simulink model "motor_sim"  (R2024a)
settings: Solver=FixedStepAuto  StartTime=0.0  StopTime=inf  FixedStep=0.0005  RelTol=1e-3
undefined symbols (not defined in the file or in its folder): B, circumference_tyre, J, K_b, K_t, L, PI, R, ratio_reduction, tau_L
libraries: canoelib x4
settings Model: Creator=user  LastModifiedBy=user

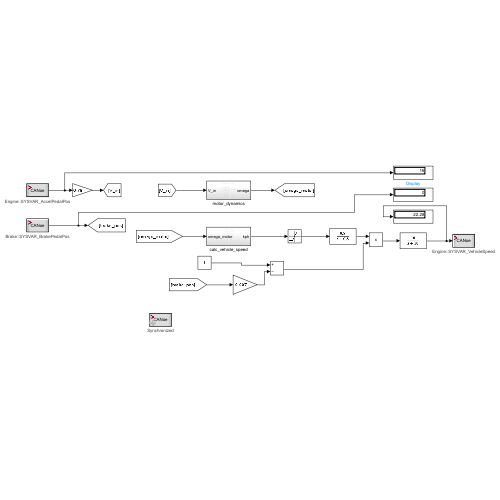
[thumbnail: Simulink's stored preview of the top-level diagram]
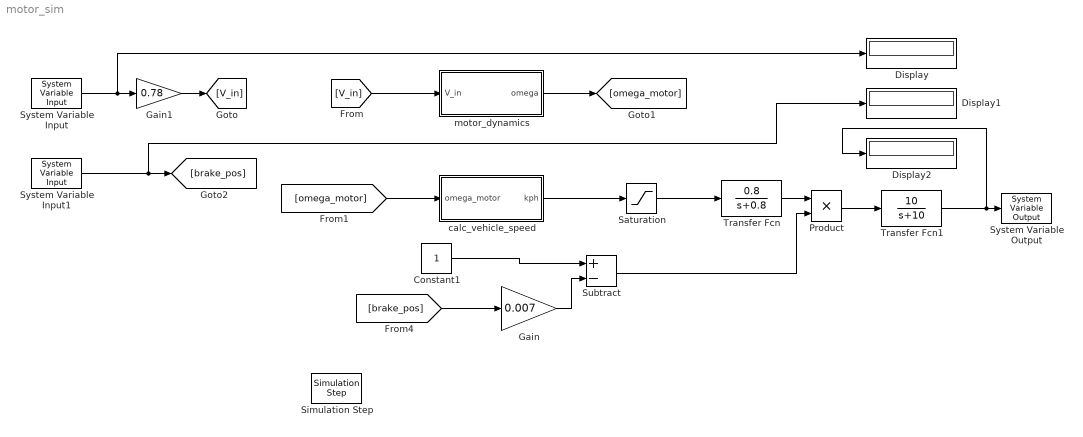
== system motor_sim ==
  Constant1 : Constant
  Display : Display
  Display1 : Display
  Display2 : Display
  Gain : Gain  Gain=0.007
  Gain1 : Gain  Gain=0.78
  Product : Product
  Saturation : Saturate  UpperLimit=250  LowerLimit=0
  Simulation Step : canoelib/CANoe I//O/Simulation Step  mode=Synchronized
      settings: AttributesFormatString=%<mode>  SourceProductName=Vector CANoe
  Subtract : Sum  Inputs=+-
  System Variable Input : canoelib/CANoe I//O/System Variable Input  nsName=Engine  sysVarName=SYSVAR_AccelPedalPos  arrayIndex=-1  editSampleTime=0  rawValue=Default  dataType=Default  dataTypeDB=uint32  hasEncoding=off  dataTypeCANoe=Get from CANoe
      settings: AttributesFormatString=%<nsName>::%<sysVarName>  SourceProductName=Vector CANoe
  System Variable Input1 : canoelib/CANoe I//O/System Variable Input  nsName=Brake  sysVarName=SYSVAR_BrakePedalPos  arrayIndex=-1  editSampleTime=0  rawValue=Default  dataType=Default  dataTypeDB=uint32  hasEncoding=off  dataTypeCANoe=Get from CANoe
      settings: AttributesFormatString=%<nsName>::%<sysVarName>  SourceProductName=Vector CANoe
  System Variable Output : canoelib/CANoe I//O/System Variable Output  nsName=Engine  sysVarName=SYSVAR_VehicleSpeed  arrayIndex=-1  rawValue=Default  dataType=Default  dataTypeDB=uint32  hasEncoding=off  dataTypeCANoe=Get from CANoe
      settings: AttributesFormatString=%<nsName>::%<sysVarName>  SourceProductName=Vector CANoe
  Transfer Fcn : TransferFcn  Numerator=[0.8]  Denominator=[1 0.8]
  Transfer Fcn1 : TransferFcn  Numerator=[10]  Denominator=[1 10]
  calc_vehicle_speed : Subsystem
  motor_dynamics : Subsystem
  wires:
  [V_in] -> motor_dynamics/1(V_in)
  motor_dynamics/1(omega) -> [omega_motor]
  calc_vehicle_speed/1(kph) -> Saturation/1
  [omega_motor] -> calc_vehicle_speed/1(omega_motor)
  [brake_pos] -> Gain/1
  Constant1/1 -> Subtract/1
  Gain/1 -> Subtract/2
  Subtract/1 -> Product/2
  Saturation/1 -> Transfer Fcn/1
  Transfer Fcn/1 -> Product/1
  Product/1 -> Transfer Fcn1/1
  System Variable Input/1 -> Display/1, Gain1/1
  Gain1/1 -> [V_in]
  System Variable Input1/1 -> Display1/1, [brake_pos]
  Transfer Fcn1/1 -> Display2/1, System Variable Output/1

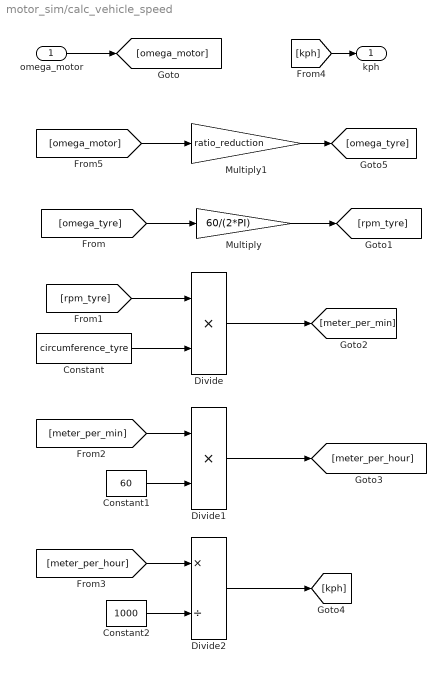
== system motor_sim/calc_vehicle_speed ==
  omega_motor : Inport
  Constant : Constant  Value=circumference_tyre
  Constant1 : Constant  Value=60
  Constant2 : Constant  Value=1000
  Divide : Product  Inputs=**
  Divide1 : Product  Inputs=**
  Divide2 : Product  Inputs=*/
  Multiply : Gain  Gain=60/(2*PI)
  Multiply1 : Gain  Gain=ratio_reduction
  kph : Outport
  wires:
  omega_motor/1 -> [omega_motor]
  [omega_tyre] -> Multiply/1
  Multiply/1 -> [rpm_tyre]
  [rpm_tyre] -> Divide/1
  Constant/1 -> Divide/2
  Divide/1 -> [meter_per_min]
  [meter_per_min] -> Divide1/1
  Constant1/1 -> Divide1/2
  Divide1/1 -> [meter_per_hour]
  [meter_per_hour] -> Divide2/1
  Constant2/1 -> Divide2/2
  Divide2/1 -> [kph]
  [kph] -> kph/1
  [omega_motor] -> Multiply1/1
  Multiply1/1 -> [omega_tyre]

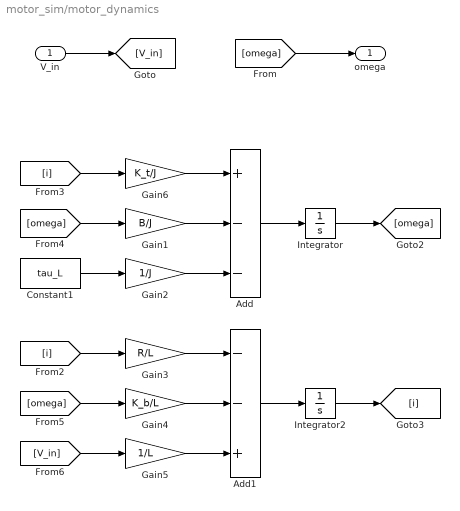
== system motor_sim/motor_dynamics ==
  V_in : Inport
  Add : Sum  Inputs=+--
  Add1 : Sum  Inputs=--+
  Constant1 : Constant  Value=tau_L
  Gain1 : Gain  Gain=B/J
  Gain2 : Gain  Gain=1/J
  Gain3 : Gain  Gain=R/L
  Gain4 : Gain  Gain=K_b/L
  Gain5 : Gain  Gain=1/L
  Gain6 : Gain  Gain=K_t/J
  Integrator : Integrator
  Integrator2 : Integrator
  omega : Outport
  wires:
  Gain5/1 -> Add1/3
  Add1/1 -> Integrator2/1
  Gain3/1 -> Add1/1
  Integrator2/1 -> [i]
  Gain6/1 -> Add/1
  [omega] -> Gain4/1
  Gain4/1 -> Add1/2
  [V_in] -> Gain5/1
  Add/1 -> Integrator/1
  Gain1/1 -> Add/2
  [i] -> Gain3/1
  Integrator/1 -> [omega]
  [i] -> Gain6/1
  Constant1/1 -> Gain2/1
  Gain2/1 -> Add/3
  [omega] -> Gain1/1
  V_in/1 -> [V_in]
  [omega] -> omega/1
